simulink model "ejemplo_cliente_hyperimu"  (R2014b)
settings: Solver=ode45  StartTime=0.0  StopTime=inf  RelTol=1e-3
libraries: LibrarySimulinkSAS x1
settings Model: Creator=labo robot  LastModifiedBy=labo robot

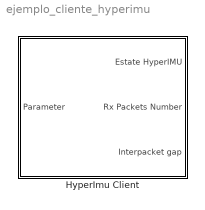
== system ejemplo_cliente_hyperimu ==
  HyperImu Client : Subsystem  mask{dev=1}
      mask prompts: dev "Device Number"
      mask Help:
      | HELP DEVICE
      | 
      | - UDP Client for the server "HyperIMU"-Android App
      | 
      | HELP DRIVERS
      | 
      | Install in your phone the app "HyperIMU" for Android. Link: https://play.google.com/store/apps/details?id=com.ianovir.hyper_imu&hl=es
      | -------------------------------------------------------------------------------------------------------------------------------------------------------
      | HELP APP
      | 
      | Before running the Simulink model initiate communication with the device through the application 'imu.exe' available from folder '\SAS TOOLS\Software imu V1.1.0'. After executing the program the app icon is available in the taskbar.
      | The app "HyperIMU.exe" is handled from right-click on the icon and selecting the corresponding option:
      | "Play" -> Start the commnunication between the device and the app
      | "Stop" -> Stop the communication
      | "Monitor"->view the state of sensors and communication
      | 
      | -------------------------------------------------------------------------------------------------------------------------------------------------------
      | 
      | HELP BLOCK
      | 
      | Input Ports
      | 
      | Port 'Parameters' scalar non-used.
      | 
      | Output Ports
      | 
      | Port 'State': sensors information chosen with the App HyperIMU
      | 
      | 'Rx Packets Number' number of received packets by the client
      | 
      | 'Interpacket gap' time between packets
      | 
      | -------------------------------------------------------------------------------------------------------------------------------------------------------
      | 
      | HELP SHARE MEMORY (information only for external applications different to "HyperIMU.exe")
      | 
      | Shared Memory Names:
      | 
      | 'HYPERIMU_entrada_'#dev
      | 'HYPERIMU_salida_'#dev
      | NOTE: replace #dev with the device number
      mask DialogControl DescGroupVar Prompt: HyperIMU client
      mask DialogControl DescTextVar Prompt: This block is used to receive data via UDP from the App "HyperIMU" through the application 'HyperIMU.exe' available on folder '\SAS TOOLS\Software HyperIMU V1.1.0'. More information in Help button.
      mask Display:
      | image('Client.png')
      | color('red')
      | port_label('input',1,'Parameter')
      | color('blue')
      | port_label('output',1,'Sensors')
      | port_label('output',2,'Rx Packets Number')
      | port_label('output',3,'Interpacket gap')

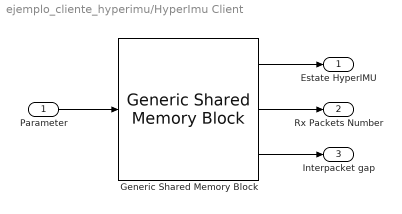
== system ejemplo_cliente_hyperimu/HyperImu Client ==
  Parameter : Inport
  Generic Shared Memory Block : LibrarySimulinkSAS/Generic Shared Memory Block  nombre='HYPERIMU'  dispositivo=dev  vecE=[1]  vecS=[12 1 1]  tipoE=['f']  tipoS=['f' 'I' 'f']
  Estate HyperIMU : Outport
  Rx Packets Number : Outport  Port=2
  Interpacket gap : Outport  Port=3
  wires:
  Generic Shared Memory Block/2 -> Rx Packets Number/1
  Generic Shared Memory Block/3 -> Interpacket gap/1
  Generic Shared Memory Block/1 -> Estate HyperIMU/1
  Parameter/1 -> Generic Shared Memory Block/1
